simulink model "G2V"  (R2017a)
settings: Solver=ode23t  StartTime=0.0  StopTime=10  RelTol=1e-3
values from neighbouring files (symbols this model uses):
  C_Vdc = 100*18e-3    (= 1.8)    [main_v2gg2v.m]
  Cf = 10*165e-6    (= 0.00165)    [main_v2gg2v.m]
  D = 20    [main_v2gg2v.m]
  E1 = 1.07364213042869    (= 1.07364213043)    [main_v2gg2v.m]
  E2 = 1.05726676017896    (= 1.05726676018)    [main_v2gg2v.m]
  E3 = 1.05298913370226    (= 1.0529891337)    [main_v2gg2v.m]
  f_grid = 50    [main_v2gg2v.m]
  H1 = 10    [main_v2gg2v.m]
  H2 = 15    [main_v2gg2v.m]
  H3 = 60    [main_v2gg2v.m]
  h_PEV = -2000    [main_v2gg2v.m]
  Ibat_ref = -200    [main_v2gg2v.m]
  Ibatfault_ref = 200    [main_v2gg2v.m]
  Ki_CC = 1    [main_v2gg2v.m]
  Ki_inner = 5000    [main_v2gg2v.m]
  Ki_outer = 10000    [main_v2gg2v.m]
  Ki_PLL = 10000    [main_v2gg2v.m]
  Kp_CC = 10    [main_v2gg2v.m]
  Kp_inner = 100    [main_v2gg2v.m]
  Kp_outer = 250    [main_v2gg2v.m]
  Kp_PLL = 100    [main_v2gg2v.m]
  Lbat = 2e-3    (= 0.002)    [main_v2gg2v.m]
  Lgrid = 1/10*0.69e-3    (= 6.9e-05)    [main_v2gg2v.m]
  Linv = 1/10*0.48e-3    (= 4.8e-05)    [main_v2gg2v.m]
  LowSat_CC = 0    [main_v2gg2v.m]
  omega = 2*pi*f_grid    (= 314.159265359)    [main_v2gg2v.m]
  Pm1 = 2.49    [main_v2gg2v.m]
  Pm2 = 4.21    [main_v2gg2v.m]
  Pm3 = 8.20    (= 8.2)    [main_v2gg2v.m]
  Rd = 1.31    [main_v2gg2v.m]
  S1pu = (1.5 + .45j)    [main_v2gg2v.m]
  S2pu = (1.0 + .3j)    [main_v2gg2v.m]
  S3pu = (12.4 + 2.5j)    [main_v2gg2v.m]
  Sbase = 1e6    (= 1000000)    [main_v2gg2v.m]
  Snom_trafo = 1050e6    (= 1050000000)    [main_v2gg2v.m]
  t_fault_end = t_fault_start + FCT    (= 0.723)    [main_v2gg2v.m]
  t_fault_start = 0.5    [main_v2gg2v.m]
  Ts = 1e-5    (= 1e-05)    [main_v2gg2v.m]
  UpSat_CC = 1    [main_v2gg2v.m]
  Vbase = 345e3    (= 345000)    [main_v2gg2v.m]
  Vdc_ref = 1.5e3    (= 1500)    [main_v2gg2v.m]
  Vfault_thresh = 455    [main_v2gg2v.m]
undefined symbols (not defined in the file or in its folder): D1, Delta, Ion, L12, L13, L23, Lbuckboost, Lithium, R_Vdc, Rbuckboost
libraries: powerlib x175, powerlib_meascontrol x55, simulink x45, electricdrivelib x30, dspstat3 x3
(part 1 of 5)
settings Model: Creator=BagaskaraPP  LastModifiedBy=BagaskaraPP
settings SolverCC: ZeroCrossAlgorithm=Adaptive
settings DataIOCC: Refine=4
settings DebuggingCC: MaxConsecutiveZCsMsg=none

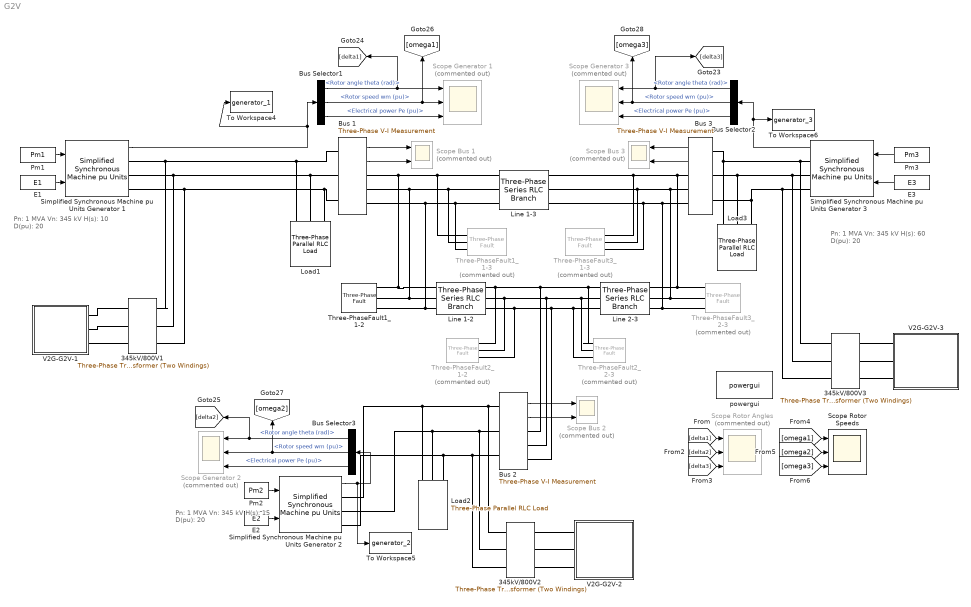
== system G2V ==
  note: Pn: 1 MVA
      | Vn: 345 kV
      | H(s): 15
      | D(pu): 20
  note: Pn: 1 MVA
      | Vn: 345 kV
      | H(s): 60
      | D(pu): 20
  note: Pn: 1 MVA
      | Vn: 345 kV
      | H(s): 10
      | D(pu): 20
  345kV/800V1 : powerlib/Elements/Three-Phase Transformer (Two Windings)  Winding1Connection=Delta (D1)  Winding2Connection=Yg  CoreType=Three single-phase transformers  SetSaturation=off  Hysteresis=off  DataFile='hysteresis'  SetInitialFlux=off  Measurements=None  UNITS=pu  NominalPower=[ Snom_trafo , f_grid ]  Winding1=[Vbase , 0 , 0 ]  Winding2=[ 800 , 0 , 0 ]  Rm=0  Lm=0  L0=0.5  Saturation=[ 0,0 ; 0.0024,1.2 ; 1.0,1.52 ]  InitialFluxes=[ 0.8 , -0.8 , 0.7 ]  MoreParameters=off  BreakLoop=off  DataType=off  TransfoNumber=1
  345kV/800V2 : powerlib/Elements/Three-Phase Transformer (Two Windings)  Winding1Connection=Delta (D1)  Winding2Connection=Yg  CoreType=Three single-phase transformers  SetSaturation=off  Hysteresis=off  DataFile='hysteresis'  SetInitialFlux=off  Measurements=None  UNITS=pu  NominalPower=[ Snom_trafo , f_grid ]  Winding1=[Vbase , 0 , 0 ]  Winding2=[ 800 , 0 , 0 ]  Rm=0  Lm=0  L0=0.5  Saturation=[ 0,0 ; 0.0024,1.2 ; 1.0,1.52 ]  InitialFluxes=[ 0.8 , -0.8 , 0.7 ]  MoreParameters=off  BreakLoop=off  DataType=off  TransfoNumber=1
  345kV/800V3 : powerlib/Elements/Three-Phase Transformer (Two Windings)  Winding1Connection=Delta (D1)  Winding2Connection=Yg  CoreType=Three single-phase transformers  SetSaturation=off  Hysteresis=off  DataFile='hysteresis'  SetInitialFlux=off  Measurements=None  UNITS=pu  NominalPower=[ Snom_trafo , f_grid ]  Winding1=[Vbase , 0 , 0 ]  Winding2=[ 800 , 0 , 0 ]  Rm=0  Lm=0  L0=0.5  Saturation=[ 0,0 ; 0.0024,1.2 ; 1.0,1.52 ]  InitialFluxes=[ 0.8 , -0.8 , 0.7 ]  MoreParameters=off  BreakLoop=off  DataType=off  TransfoNumber=1
  Bus Selector1 : BusSelector  OutputSignals=Rotor angle theta (rad),Rotor speed wm (pu),Electrical power Pe (pu)
  Bus Selector2 : BusSelector  OutputSignals=Rotor angle theta (rad),Rotor speed wm (pu),Electrical power Pe (pu)
  Bus Selector3 : BusSelector  OutputSignals=Rotor angle theta (rad),Rotor speed wm (pu),Electrical power Pe (pu)
  Bus 1 : powerlib/Measurements/Three-Phase V-I Measurement  VoltageMeasurement=phase-to-ground  SetLabelV=off  LabelV=Vabc  Vpu=off  VpuLL=off  CurrentMeasurement=yes  SetLabelI=off  LabelI=Iabc  Ipu=off  Pbase=100e6  Vbase=500e3  OutputType=Complex  PhasorSimulation=off  PSBequivalent=0
  Bus 2 : powerlib/Measurements/Three-Phase V-I Measurement  VoltageMeasurement=phase-to-ground  SetLabelV=off  LabelV=Vabc  Vpu=off  VpuLL=off  CurrentMeasurement=yes  SetLabelI=off  LabelI=Iabc  Ipu=off  Pbase=100e6  Vbase=500e3  OutputType=Complex  PhasorSimulation=off  PSBequivalent=0
  Bus 3 : powerlib/Measurements/Three-Phase V-I Measurement  VoltageMeasurement=phase-to-ground  SetLabelV=off  LabelV=Vabc  Vpu=off  VpuLL=off  CurrentMeasurement=yes  SetLabelI=off  LabelI=Iabc  Ipu=off  Pbase=100e6  Vbase=500e3  OutputType=Complex  PhasorSimulation=off  PSBequivalent=0
  E1 : Constant  Value=E1
  E2 : Constant  Value=E2
  E3 : Constant  Value=E3
  Line 1-2 : powerlib/Elements/Three-Phase Series RLC Branch  LConnTagsString=A|B|C  RConnTagsString=A|B|C  BranchType=RL  Resistance=0  Inductance=L12  Capacitance=1e-6  Measurements=None
  Line 1-3 : powerlib/Elements/Three-Phase Series RLC Branch  LConnTagsString=A|B|C  RConnTagsString=A|B|C  BranchType=RL  Resistance=0  Inductance=L13  Capacitance=1e-6  Measurements=None
  Line 2-3 : powerlib/Elements/Three-Phase Series RLC Branch  LConnTagsString=A|B|C  RConnTagsString=A|B|C  BranchType=RL  Resistance=0  Inductance=L23  Capacitance=1e-6  Measurements=None
  Load1 : powerlib/Elements/Three-Phase Parallel RLC Load  LConnTagsString=A|B|C  Configuration=Y (grounded)  NominalVoltage=Vbase  Vabc=[1e3 1e3 1e3]  Vabcp=[1e3 1e3 1e3]  NominalFrequency=f_grid  UnbalancedPower=off  ActivePower=real(S1pu)*Sbase  InductivePower=imag(S1pu)*Sbase  CapacitivePower=0  Pabc=[10e3 9e3 11e3]  QLabc=[100 90 110]  QCabc=[100 90 110]  Pabcp=[10e3 9e3 11e3]  QLabcp=[100 90 110]  QCabcp=[100 90 110]  Measurements=None  LoadType=constant PQ
  Load2 : powerlib/Elements/Three-Phase Parallel RLC Load  LConnTagsString=A|B|C  Configuration=Y (grounded)  NominalVoltage=Vbase  Vabc=[1e3 1e3 1e3]  Vabcp=[1e3 1e3 1e3]  NominalFrequency=f_grid  UnbalancedPower=off  ActivePower=real(S2pu)*Sbase  InductivePower=imag(S2pu)*Sbase  CapacitivePower=0  Pabc=[10e3 9e3 11e3]  QLabc=[100 90 110]  QCabc=[100 90 110]  Pabcp=[10e3 9e3 11e3]  QLabcp=[100 90 110]  QCabcp=[100 90 110]  Measurements=None  LoadType=constant PQ
  Load3 : powerlib/Elements/Three-Phase Parallel RLC Load  LConnTagsString=A|B|C  Configuration=Y (grounded)  NominalVoltage=Vbase  Vabc=[1e3 1e3 1e3]  Vabcp=[1e3 1e3 1e3]  NominalFrequency=f_grid  UnbalancedPower=off  ActivePower=real(S3pu)*Sbase  InductivePower=imag(S3pu)*Sbase  CapacitivePower=0  Pabc=[10e3 9e3 11e3]  QLabc=[100 90 110]  QCabc=[100 90 110]  Pabcp=[10e3 9e3 11e3]  QLabcp=[100 90 110]  QCabcp=[100 90 110]  Measurements=None  LoadType=constant PQ
  Pm1 : Constant  Value=Pm1
  Pm2 : Constant  Value=Pm2
  Pm3 : Constant  Value=Pm3
  Scope Bus 1 : Scope  Commented=on  NumInputPorts=2
  Scope Bus 2 : Scope  Commented=on  NumInputPorts=2
  Scope Bus 3 : Scope  Commented=on  NumInputPorts=2
  Scope Generator 1 : Scope  Commented=on  NumInputPorts=3
  Scope Generator 2 : Scope  Commented=on  NumInputPorts=3
  Scope Generator 3 : Scope  Commented=on  NumInputPorts=3
  Scope Rotor Angles : Scope  Commented=on  NumInputPorts=3
  Scope Rotor Speeds : Scope  NumInputPorts=3
  Simplified Synchronous Machine pu Units Generator 1 : powerlib/Machines/Simplified Synchronous Machine pu Units  ConnectionType=3-wire Y  MechanicalLoad=Mechanical power Pm  MeasurementBus=off  NominalParameters=[Sbase Vbase f_grid]  Mechanical=[H1 D 1]  InternalRL="[0.0  0.088]"  InitialConditions="[ 0,26.7181   2.5567,2.5567,2.5567   15,15-120,15+120 ]"  Units=0  LoadFlowParameters=[1,0,0,0,0]  TsPowergui=0  TsBlock=-1  BusType=PV  Pref=0  Qref=0  Qmin=-inf  Qmax=+inf  PLF=0  QLF=0
      settings: SourceProductName=Simscape Power Systems  SourceProductBaseCode=PS
  Simplified Synchronous Machine pu Units Generator 2 : powerlib/Machines/Simplified Synchronous Machine pu Units  ConnectionType=3-wire Y  MechanicalLoad=Mechanical power Pm  MeasurementBus=off  NominalParameters=[Sbase Vbase f_grid]  Mechanical=[H2 D 1]  InternalRL="[0.0  0.05]"  InitialConditions="[ 0,26.4706   4.2715,4.2715,4.2715   15,15-120,15+120 ]"  Units=0  LoadFlowParameters=[1,0,0,0,0]  TsPowergui=0  TsBlock=-1  BusType=PV  Pref=0  Qref=0  Qmin=-inf  Qmax=+inf  PLF=0  QLF=0
      settings: SourceProductName=Simscape Power Systems  SourceProductBaseCode=PS
  Simplified Synchronous Machine pu Units Generator 3 : powerlib/Machines/Simplified Synchronous Machine pu Units  ConnectionType=3-wire Y  MechanicalLoad=Mechanical power Pm  MeasurementBus=off  NominalParameters=[Sbase Vbase f_grid]  Mechanical=[H3 D 1]  InternalRL="[0.0  0.015]"  InitialConditions="[ 0,6.7081   8.7496,8.7496,8.7496   0,-120,120 ]"  Units=0  LoadFlowParameters=[1,0,0,0,0]  TsPowergui=0  TsBlock=-1  BusType=PV  Pref=0  Qref=0  Qmin=-inf  Qmax=+inf  PLF=0  QLF=0
      settings: SourceProductName=Simscape Power Systems  SourceProductBaseCode=PS
  Three-PhaseFault1_1-2 : powerlib/Elements/Three-Phase Fault  InitialStates=0  FaultA=on  FaultB=on  FaultC=on  GroundFault=on  SwitchTimes="[t_fault_start  t_fault_end]"  External=off  SwitchStatus=NaN  FaultResistance=0.001  GroundResistance=0.01  SnubberResistance=1e6  SnubberCapacitance=inf  Measurements=None
  Three-PhaseFault1_1-3 : powerlib/Elements/Three-Phase Fault  Commented=on  InitialStates=0  FaultA=on  FaultB=on  FaultC=on  GroundFault=on  SwitchTimes="[t_fault_start  t_fault_end]"  External=off  SwitchStatus=NaN  FaultResistance=0.001  GroundResistance=0.01  SnubberResistance=1e6  SnubberCapacitance=inf  Measurements=None
  Three-PhaseFault2_1-2 : powerlib/Elements/Three-Phase Fault  Commented=on  InitialStates=0  FaultA=on  FaultB=on  FaultC=on  GroundFault=on  SwitchTimes="[t_fault_start  t_fault_end]"  External=off  SwitchStatus=NaN  FaultResistance=0.001  GroundResistance=0.01  SnubberResistance=1e6  SnubberCapacitance=inf  Measurements=None
  Three-PhaseFault2_2-3 : powerlib/Elements/Three-Phase Fault  Commented=on  InitialStates=0  FaultA=on  FaultB=on  FaultC=on  GroundFault=on  SwitchTimes="[t_fault_start  t_fault_end]"  External=off  SwitchStatus=NaN  FaultResistance=0.001  GroundResistance=0.01  SnubberResistance=1e6  SnubberCapacitance=inf  Measurements=None
  Three-PhaseFault3_1-3 : powerlib/Elements/Three-Phase Fault  Commented=on  InitialStates=0  FaultA=on  FaultB=on  FaultC=on  GroundFault=on  SwitchTimes="[t_fault_start  t_fault_end]"  External=off  SwitchStatus=NaN  FaultResistance=0.001  GroundResistance=0.01  SnubberResistance=1e6  SnubberCapacitance=inf  Measurements=None
  Three-PhaseFault3_2-3 : powerlib/Elements/Three-Phase Fault  Commented=on  InitialStates=0  FaultA=on  FaultB=on  FaultC=on  GroundFault=on  SwitchTimes="[t_fault_start  t_fault_end]"  External=off  SwitchStatus=NaN  FaultResistance=0.001  GroundResistance=0.01  SnubberResistance=1e6  SnubberCapacitance=inf  Measurements=None
  To Workspace4 : ToWorkspace  VariableName=generator_1  SaveFormat=Timeseries  SampleTime=-1
  To Workspace5 : ToWorkspace  VariableName=generator_2  SaveFormat=Timeseries  SampleTime=-1
  To Workspace6 : ToWorkspace  VariableName=generator_3  SaveFormat=Timeseries  SampleTime=-1
  V2G-G2V-1 : Subsystem
  V2G-G2V-2 : Subsystem
  V2G-G2V-3 : Subsystem
  powergui : powerlib/powergui  Priority=1  SimulationMode=Discrete  SampleTime=Ts  frequency=60  Iterations=50  frequencyindice=0  Pbase=100e6  ErrMax=1e-4  UnitsV=kV  UnitsW=MW  buscounter=0  FunctionMessages=off  echomessages=off  EnableUseOfTLC=off  CurrentSourceSwitches=off  DisableSnubberDevices=off  DisableRonSwitches=off  DisableVfSwitches=off  DisplayEquations=off  SolverType=Tustin/Backward Euler (TBE)  Interpol=off  ExternalGateDelay=off  methode=off  Ts=100  x0status=blocks  SPID=on  SwTol=0  HookPort=off  RestoreLinks=warning  ResistiveCurrentMeasurement=off  Frange=[0:2:500]  Ylog=off  Xlog=on  ShowGrid=off  save=off  variable=ZData  structure=0  ZoomFFT=off  StartTime=0.0  cycles=1  DisplayStyle=1  fundamental=60  FreqAxis=off  MaxFrequency=1000  frequencyindicesteady=1  RmsSteady=1  display=off
  wires:
  Bus 1/1 -> Scope Bus 1/1
  Pm2/1 -> Simplified Synchronous Machine pu Units Generator 2/1
  Bus Selector2/2 -> [omega3], Scope Generator 3/2  "<Rotor speed wm (pu)>"
  Bus Selector2/1 -> Scope Generator 3/1, [delta3]  "<Rotor angle theta (rad)>"
  Pm3/1 -> Simplified Synchronous Machine pu Units Generator 3/1
  Bus 2/2 -> Scope Bus 2/2
  Bus Selector3/3 -> Scope Generator 2/3  "<Electrical power Pe (pu)>"
  Bus Selector2/3 -> Scope Generator 3/3  "<Electrical power Pe (pu)>"
  Bus 1/2 -> Scope Bus 1/2
  Bus Selector3/2 -> Scope Generator 2/2, [omega2]  "<Rotor speed wm (pu)>"
  Bus 3/2 -> Scope Bus 3/2
  Bus Selector3/1 -> Scope Generator 2/1, [delta2]  "<Rotor angle theta (rad)>"
  Bus 3/1 -> Scope Bus 3/1
  Bus 2/1 -> Scope Bus 2/1
  E1/1 -> Simplified Synchronous Machine pu Units Generator 1/2
  Pm1/1 -> Simplified Synchronous Machine pu Units Generator 1/1
  Simplified Synchronous Machine pu Units Generator 1/1 -> To Workspace4/1, Bus Selector1/1
  Bus Selector1/3 -> Scope Generator 1/3  "<Electrical power Pe (pu)>"
  Simplified Synchronous Machine pu Units Generator 3/1 -> To Workspace6/1, Bus Selector2/1
  Bus Selector1/2 -> Scope Generator 1/2, [omega1]  "<Rotor speed wm (pu)>"
  Bus Selector1/1 -> Scope Generator 1/1, [delta1]  "<Rotor angle theta (rad)>"
  Simplified Synchronous Machine pu Units Generator 2/1 -> To Workspace5/1, Bus Selector3/1
  E2/1 -> Simplified Synchronous Machine pu Units Generator 2/2
  E3/1 -> Simplified Synchronous Machine pu Units Generator 3/2
  [omega2] -> Scope Rotor Speeds/2
  [delta2] -> Scope Rotor Angles/2
  [delta3] -> Scope Rotor Angles/3
  [delta1] -> Scope Rotor Angles/1
  [omega3] -> Scope Rotor Speeds/3
  [omega1] -> Scope Rotor Speeds/1
  connections:
  Line 1-2/LConn1 -- Three-PhaseFault1_1-2/LConn1 -- Three-PhaseFault1_1-3/LConn1 -- Line 1-3/LConn1 -- Bus 1/RConn1
  Load1/LConn3 -- 345kV/800V1/LConn3 -- Simplified Synchronous Machine pu Units Generator 1/RConn3 -- Bus 1/LConn3
  Three-PhaseFault2_1-2/LConn2 -- Line 1-2/RConn2 -- Bus 2/RConn2 -- Three-PhaseFault2_2-3/LConn2 -- Line 2-3/LConn2
  Load3/LConn3 -- 345kV/800V3/LConn3 -- Simplified Synchronous Machine pu Units Generator 3/RConn3 -- Bus 3/LConn3
  Load2/LConn2 -- 345kV/800V2/LConn2 -- Bus 2/LConn2 -- Simplified Synchronous Machine pu Units Generator 2/RConn2
  Bus 3/RConn2 -- Three-PhaseFault3_2-3/LConn2 -- Line 2-3/RConn2 -- Line 1-3/RConn2 -- Three-PhaseFault3_1-3/LConn2
  Bus 3/RConn3 -- Three-PhaseFault3_2-3/LConn3 -- Line 2-3/RConn3 -- Line 1-3/RConn3 -- Three-PhaseFault3_1-3/LConn3
  Load1/LConn2 -- 345kV/800V1/LConn2 -- Simplified Synchronous Machine pu Units Generator 1/RConn2 -- Bus 1/LConn2
  Simplified Synchronous Machine pu Units Generator 2/RConn1 -- Load2/LConn1 -- 345kV/800V2/LConn1 -- Bus 2/LConn1
  Load3/LConn1 -- 345kV/800V3/LConn1 -- Simplified Synchronous Machine pu Units Generator 3/RConn1 -- Bus 3/LConn1
  Line 2-3/LConn1 -- Three-PhaseFault2_2-3/LConn1 -- Bus 2/RConn1 -- Three-PhaseFault2_1-2/LConn1 -- Line 1-2/RConn1
  Load3/LConn2 -- 345kV/800V3/LConn2 -- Simplified Synchronous Machine pu Units Generator 3/RConn2 -- Bus 3/LConn2
  Line 1-3/RConn1 -- Three-PhaseFault3_1-3/LConn1 -- Three-PhaseFault3_2-3/LConn1 -- Line 2-3/RConn1 -- Bus 3/RConn1
  Load2/LConn3 -- Simplified Synchronous Machine pu Units Generator 2/RConn3 -- 345kV/800V2/LConn3 -- Bus 2/LConn3
  Line 1-3/LConn2 -- Three-PhaseFault1_1-3/LConn2 -- Line 1-2/LConn2 -- Three-PhaseFault1_1-2/LConn2 -- Bus 1/RConn2
  Line 1-2/LConn3 -- Three-PhaseFault1_1-3/LConn3 -- Line 1-3/LConn3 -- Bus 1/RConn3 -- Three-PhaseFault1_1-2/LConn3
  Bus 1/LConn1 -- 345kV/800V1/LConn1 -- Simplified Synchronous Machine pu Units Generator 1/RConn1 -- Load1/LConn1
  Three-PhaseFault2_1-2/LConn3 -- Line 1-2/RConn3 -- Bus 2/RConn3 -- Three-PhaseFault2_2-3/LConn3 -- Line 2-3/LConn3
  345kV/800V2/RConn1 -- V2G-G2V-2/LConn1
  345kV/800V2/RConn2 -- V2G-G2V-2/LConn2
  345kV/800V2/RConn3 -- V2G-G2V-2/LConn3
  V2G-G2V-1/LConn1 -- 345kV/800V1/RConn1
  V2G-G2V-1/LConn2 -- 345kV/800V1/RConn2
  V2G-G2V-1/LConn3 -- 345kV/800V1/RConn3
  V2G-G2V-3/LConn1 -- 345kV/800V3/RConn1
  V2G-G2V-3/LConn2 -- 345kV/800V3/RConn2
  V2G-G2V-3/LConn3 -- 345kV/800V3/RConn3

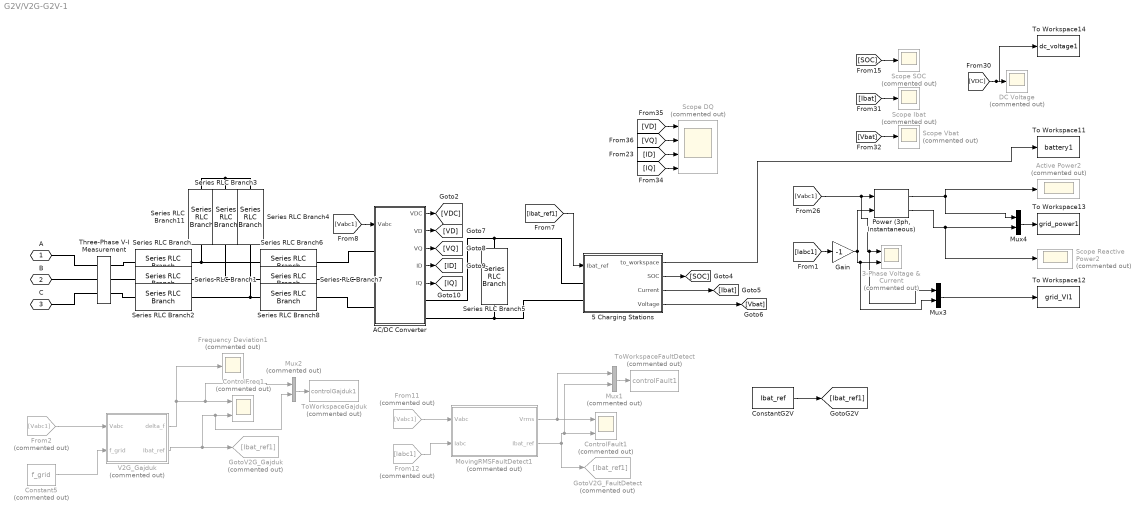
== system G2V/V2G-G2V-1 ==
  3-Phase Voltage & Current : Scope  Commented=on  NumInputPorts=2
  5 Charging Stations : Subsystem
  AC/DC Converter : Subsystem
  Active Power2 : Scope  Commented=on
  Constant5 : Constant  Commented=on  Value=f_grid
  ConstantG2V : Constant  Value=Ibat_ref
  ControlFault1 : Scope  Commented=on  NumInputPorts=2
  ControlFreq1 : Scope  Commented=on  NumInputPorts=2
  DC Voltage : Scope  Commented=on
  Frequency Deviation1 : Scope  Commented=on
  From11 : From  Commented=on  GotoTag=Vabc1  TagVisibility=global
  From12 : From  Commented=on  GotoTag=Iabc1  TagVisibility=global
  From2 : From  Commented=on  GotoTag=Vabc1  TagVisibility=global
  Gain : Gain  Gain=-1
  GotoV2G_FaultDetect : Goto  Commented=on  GotoTag=Ibat_ref1
  GotoV2G_Gajduk : Goto  Commented=on  GotoTag=Ibat_ref1
  MovingRMSFaultDetect1 : Subsystem  Commented=on
  Mux1 : Mux  Commented=on  Inputs=2
  Mux2 : Mux  Commented=on  Inputs=2
  Mux3 : Mux  Inputs=2
  Mux4 : Mux  Inputs=2
  "Power (3ph, Instantaneous)" : powerlib_meascontrol/Measurements/Power (3ph, Instantaneous)
      settings: SourceProductName=Simscape Power Systems
  Scope DQ : Scope  Commented=on  NumInputPorts=4
  Scope Ibat : Scope  Commented=on
  Scope Reactive Power2 : Scope  Commented=on
  Scope SOC : Scope  Commented=on
  Scope Vbat : Scope  Commented=on
  Series RLC Branch : powerlib/Elements/Series RLC Branch  LConnTagsString=__new0  RConnTagsString=__new0  BranchType=L  Resistance=1  Inductance=Lgrid  SetiL0=off  InitialCurrent=0  Capacitance=1e-6  Setx0=off  InitialVoltage=0  Measurements=None
  Series RLC Branch1 : powerlib/Elements/Series RLC Branch  LConnTagsString=__new0  RConnTagsString=__new0  BranchType=L  Resistance=1  Inductance=Lgrid  SetiL0=off  InitialCurrent=0  Capacitance=1e-6  Setx0=off  InitialVoltage=0  Measurements=None
  Series RLC Branch11 : powerlib/Elements/Series RLC Branch  LConnTagsString=__new0  RConnTagsString=__new0  BranchType=RC  Resistance=Rd  Inductance=Lbuckboost  SetiL0=off  InitialCurrent=0  Capacitance=Cf  Setx0=off  InitialVoltage=0  Measurements=None
  Series RLC Branch2 : powerlib/Elements/Series RLC Branch  LConnTagsString=__new0  RConnTagsString=__new0  BranchType=L  Resistance=1  Inductance=Lgrid  SetiL0=off  InitialCurrent=0  Capacitance=1e-6  Setx0=off  InitialVoltage=0  Measurements=None
  Series RLC Branch3 : powerlib/Elements/Series RLC Branch  LConnTagsString=__new0  RConnTagsString=__new0  BranchType=RC  Resistance=Rd  Inductance=Lbuckboost  SetiL0=off  InitialCurrent=0  Capacitance=Cf  Setx0=off  InitialVoltage=0  Measurements=None
  Series RLC Branch4 : powerlib/Elements/Series RLC Branch  LConnTagsString=__new0  RConnTagsString=__new0  BranchType=RC  Resistance=Rd  Inductance=Lbuckboost  SetiL0=off  InitialCurrent=0  Capacitance=Cf  Setx0=off  InitialVoltage=0  Measurements=None
  Series RLC Branch5 : powerlib/Elements/Series RLC Branch  LConnTagsString=__new0  RConnTagsString=__new0  BranchType=C  Resistance=R_Vdc  Inductance=1e-3  SetiL0=off  InitialCurrent=0  Capacitance=C_Vdc  Setx0=on  InitialVoltage=V0_Vdc  Measurements=None
  Series RLC Branch6 : powerlib/Elements/Series RLC Branch  LConnTagsString=__new0  RConnTagsString=__new0  BranchType=L  Resistance=1  Inductance=Linv  SetiL0=off  InitialCurrent=0  Capacitance=1e-6  Setx0=off  InitialVoltage=0  Measurements=None
  Series RLC Branch7 : powerlib/Elements/Series RLC Branch  LConnTagsString=__new0  RConnTagsString=__new0  BranchType=L  Resistance=1  Inductance=Linv  SetiL0=off  InitialCurrent=0  Capacitance=1e-6  Setx0=off  InitialVoltage=0  Measurements=None
  Series RLC Branch8 : powerlib/Elements/Series RLC Branch  LConnTagsString=__new0  RConnTagsString=__new0  BranchType=L  Resistance=1  Inductance=Linv  SetiL0=off  InitialCurrent=0  Capacitance=1e-6  Setx0=off  InitialVoltage=0  Measurements=None
  Three-Phase V-I Measurement : powerlib/Measurements/Three-Phase V-I Measurement  VoltageMeasurement=phase-to-ground  SetLabelV=on  LabelV=Vabc1  Vpu=off  VpuLL=off  CurrentMeasurement=yes  SetLabelI=on  LabelI=Iabc1  Ipu=off  Pbase=100e6  Vbase=500e3  OutputType=Complex  PhasorSimulation=off  PSBequivalent=0
  To Workspace11 : ToWorkspace  VariableName=battery1  SaveFormat=Timeseries  SampleTime=-1
  To Workspace12 : ToWorkspace  VariableName=grid_VI1  SaveFormat=Timeseries  SampleTime=-1
  To Workspace13 : ToWorkspace  VariableName=grid_power1  SaveFormat=Timeseries  SampleTime=-1
  To Workspace14 : ToWorkspace  VariableName=dc_voltage1  SaveFormat=Timeseries  SampleTime=-1
  ToWorkspaceFaultDetect : ToWorkspace  Commented=on  VariableName=controlFault1  SaveFormat=Timeseries  SampleTime=-1
  ToWorkspaceGajduk : ToWorkspace  Commented=on  VariableName=controlGajduk1  SaveFormat=Timeseries  SampleTime=-1
  V2G_Gajduk : Subsystem  Commented=on
  A : PMIOPort  Port=1  Side=Left
  B : PMIOPort  Port=2  Side=Left
  C : PMIOPort  Port=3  Side=Left
  wires:
  AC/DC Converter/3(VQ) -> [VQ]
  [Iabc1] -> Gain/1
  [ID] -> Scope DQ/3
  AC/DC Converter/1(VDC) -> [VDC]
  AC/DC Converter/4(ID) -> [ID]
  [Ibat] -> Scope Ibat/1
  Gain/1 -> Mux3/2, 3-Phase Voltage & Current/2, "Power (3ph, Instantaneous)"/2
  AC/DC Converter/2(VD) -> [VD]
  [IQ] -> Scope DQ/4
  [VD] -> Scope DQ/1
  [VQ] -> Scope DQ/2
  [Ibat_ref1] -> 5 Charging Stations/1(Ibat_ref)
  5 Charging Stations/2(SOC) -> [SOC]
  5 Charging Stations/3(Current) -> [Ibat]
  [Vbat] -> Scope Vbat/1
  5 Charging Stations/4(Voltage) -> [Vbat]
  [Vabc1] -> Mux3/1, 3-Phase Voltage & Current/1, "Power (3ph, Instantaneous)"/1
  AC/DC Converter/5(IQ) -> [IQ]
  [Vabc1] -> AC/DC Converter/1(Vabc)
  [SOC] -> Scope SOC/1
  Mux4/1 -> To Workspace13/1
  "Power (3ph, Instantaneous)"/2 -> Scope Reactive Power2/1, Mux4/2
  [VDC] -> To Workspace14/1, DC Voltage/1
  Mux3/1 -> To Workspace12/1
  "Power (3ph, Instantaneous)"/1 -> Mux4/1, Active Power2/1
  5 Charging Stations/1(to_workspace) -> To Workspace11/1
  V2G_Gajduk/2(Ibat_ref) -> Mux2/2, ControlFreq1/2, GotoV2G_Gajduk/1
  V2G_Gajduk/1(delta_f) -> Mux2/1, ControlFreq1/1, Frequency Deviation1/1
  Constant5/1 -> V2G_Gajduk/2(f_grid)
  Mux2/1 -> ToWorkspaceGajduk/1
  From2/1 -> V2G_Gajduk/1(Vabc)
  Mux1/1 -> ToWorkspaceFaultDetect/1
  From12/1 -> MovingRMSFaultDetect1/2(Iabc)
  MovingRMSFaultDetect1/1(Vrms) -> Mux1/1, ControlFault1/1
  From11/1 -> MovingRMSFaultDetect1/1(Vabc)
  MovingRMSFaultDetect1/2(Ibat_ref) -> Mux1/2, ControlFault1/2, GotoV2G_FaultDetect/1
  ConstantG2V/1 -> [Ibat_ref1]
  connections:
  Series RLC Branch5/LConn1 -- 5 Charging Stations/LConn1 -- AC/DC Converter/RConn1
  Series RLC Branch6/LConn1 -- Series RLC Branch11/LConn1 -- Series RLC Branch/RConn1
  Series RLC Branch4/LConn1 -- Series RLC Branch8/LConn1 -- Series RLC Branch2/RConn1
  B/RConn1 -- Three-Phase V-I Measurement/LConn2
  Series RLC Branch/LConn1 -- Three-Phase V-I Measurement/RConn1
  A/RConn1 -- Three-Phase V-I Measurement/LConn1
  AC/DC Converter/LConn1 -- Series RLC Branch6/RConn1
  AC/DC Converter/LConn3 -- Series RLC Branch8/RConn1
  Series RLC Branch3/LConn1 -- Series RLC Branch1/RConn1 -- Series RLC Branch7/LConn1
  Series RLC Branch1/LConn1 -- Three-Phase V-I Measurement/RConn2
  5 Charging Stations/LConn2 -- Series RLC Branch5/RConn1 -- AC/DC Converter/RConn2
  Series RLC Branch11/RConn1 -- Series RLC Branch4/RConn1 -- Series RLC Branch3/RConn1
  C/RConn1 -- Three-Phase V-I Measurement/LConn3
  AC/DC Converter/LConn2 -- Series RLC Branch7/RConn1
  Series RLC Branch2/LConn1 -- Three-Phase V-I Measurement/RConn3

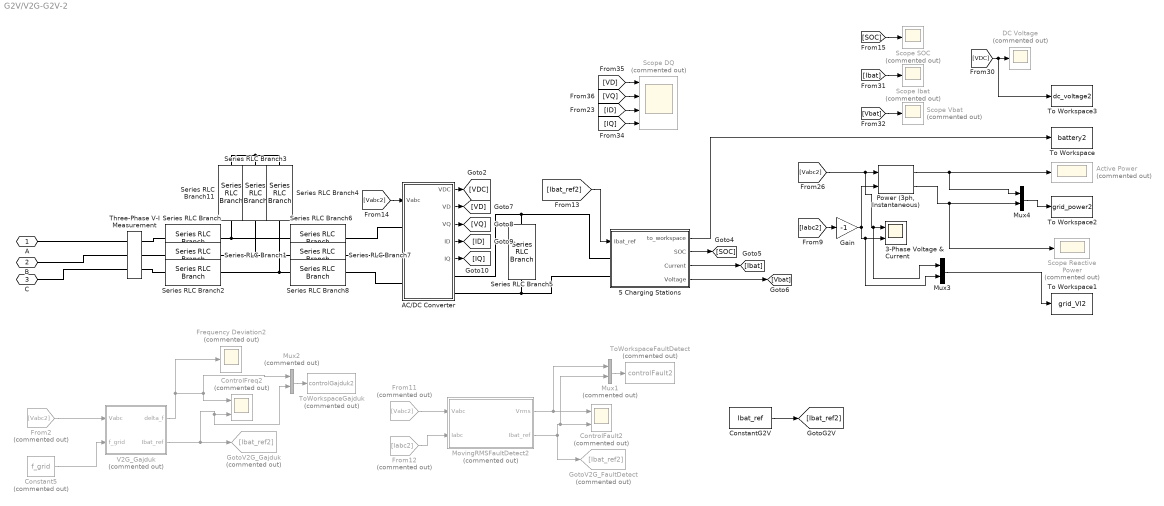
== system G2V/V2G-G2V-2 ==
  3-Phase Voltage & Current : Scope  NumInputPorts=2
  5 Charging Stations : Subsystem
  AC/DC Converter : Subsystem
  Active Power : Scope  Commented=on
  Constant5 : Constant  Commented=on  Value=f_grid
  ConstantG2V : Constant  Value=Ibat_ref
  ControlFault2 : Scope  Commented=on  NumInputPorts=2
  ControlFreq2 : Scope  Commented=on  NumInputPorts=2
  DC Voltage : Scope  Commented=on
  Frequency Deviation2 : Scope  Commented=on
  From11 : From  Commented=on  GotoTag=Vabc2  TagVisibility=global
  From12 : From  Commented=on  GotoTag=Iabc2  TagVisibility=global
  From2 : From  Commented=on  GotoTag=Vabc2  TagVisibility=global
  Gain : Gain  Gain=-1
  GotoV2G_FaultDetect : Goto  Commented=on  GotoTag=Ibat_ref2
  GotoV2G_Gajduk : Goto  Commented=on  GotoTag=Ibat_ref2
  MovingRMSFaultDetect2 : Subsystem  Commented=on
  Mux1 : Mux  Commented=on  Inputs=2
  Mux2 : Mux  Commented=on  Inputs=2
  Mux3 : Mux  Inputs=2
  Mux4 : Mux  Inputs=2
  "Power (3ph, Instantaneous)" : powerlib_meascontrol/Measurements/Power (3ph, Instantaneous)
      settings: SourceProductName=Simscape Power Systems
  Scope DQ : Scope  Commented=on  NumInputPorts=4
  Scope Ibat : Scope  Commented=on
  Scope Reactive Power : Scope  Commented=on
  Scope SOC : Scope  Commented=on
  Scope Vbat : Scope  Commented=on
  Series RLC Branch : powerlib/Elements/Series RLC Branch  LConnTagsString=__new0  RConnTagsString=__new0  BranchType=L  Resistance=1  Inductance=Lgrid  SetiL0=off  InitialCurrent=0  Capacitance=1e-6  Setx0=off  InitialVoltage=0  Measurements=None
  Series RLC Branch1 : powerlib/Elements/Series RLC Branch  LConnTagsString=__new0  RConnTagsString=__new0  BranchType=L  Resistance=1  Inductance=Lgrid  SetiL0=off  InitialCurrent=0  Capacitance=1e-6  Setx0=off  InitialVoltage=0  Measurements=None
  Series RLC Branch11 : powerlib/Elements/Series RLC Branch  LConnTagsString=__new0  RConnTagsString=__new0  BranchType=RC  Resistance=Rd  Inductance=Lbuckboost  SetiL0=off  InitialCurrent=0  Capacitance=Cf  Setx0=off  InitialVoltage=0  Measurements=None
  Series RLC Branch2 : powerlib/Elements/Series RLC Branch  LConnTagsString=__new0  RConnTagsString=__new0  BranchType=L  Resistance=1  Inductance=Lgrid  SetiL0=off  InitialCurrent=0  Capacitance=1e-6  Setx0=off  InitialVoltage=0  Measurements=None
  Series RLC Branch3 : powerlib/Elements/Series RLC Branch  LConnTagsString=__new0  RConnTagsString=__new0  BranchType=RC  Resistance=Rd  Inductance=Lbuckboost  SetiL0=off  InitialCurrent=0  Capacitance=Cf  Setx0=off  InitialVoltage=0  Measurements=None
  Series RLC Branch4 : powerlib/Elements/Series RLC Branch  LConnTagsString=__new0  RConnTagsString=__new0  BranchType=RC  Resistance=Rd  Inductance=Lbuckboost  SetiL0=off  InitialCurrent=0  Capacitance=Cf  Setx0=off  InitialVoltage=0  Measurements=None
  Series RLC Branch5 : powerlib/Elements/Series RLC Branch  LConnTagsString=__new0  RConnTagsString=__new0  BranchType=C  Resistance=R_Vdc  Inductance=1e-3  SetiL0=off  InitialCurrent=0  Capacitance=C_Vdc  Setx0=on  InitialVoltage=V0_Vdc  Measurements=None
  Series RLC Branch6 : powerlib/Elements/Series RLC Branch  LConnTagsString=__new0  RConnTagsString=__new0  BranchType=L  Resistance=1  Inductance=Linv  SetiL0=off  InitialCurrent=0  Capacitance=1e-6  Setx0=off  InitialVoltage=0  Measurements=None
  Series RLC Branch7 : powerlib/Elements/Series RLC Branch  LConnTagsString=__new0  RConnTagsString=__new0  BranchType=L  Resistance=1  Inductance=Linv  SetiL0=off  InitialCurrent=0  Capacitance=1e-6  Setx0=off  InitialVoltage=0  Measurements=None
  Series RLC Branch8 : powerlib/Elements/Series RLC Branch  LConnTagsString=__new0  RConnTagsString=__new0  BranchType=L  Resistance=1  Inductance=Linv  SetiL0=off  InitialCurrent=0  Capacitance=1e-6  Setx0=off  InitialVoltage=0  Measurements=None
  Three-Phase V-I Measurement : powerlib/Measurements/Three-Phase V-I Measurement  VoltageMeasurement=phase-to-ground  SetLabelV=on  LabelV=Vabc2  Vpu=off  VpuLL=off  CurrentMeasurement=yes  SetLabelI=on  LabelI=Iabc2  Ipu=off  Pbase=100e6  Vbase=500e3  OutputType=Complex  PhasorSimulation=off  PSBequivalent=0
  To Workspace : ToWorkspace  VariableName=battery2  SaveFormat=Timeseries  SampleTime=-1
  To Workspace1 : ToWorkspace  VariableName=grid_VI2  SaveFormat=Timeseries  SampleTime=-1
  To Workspace2 : ToWorkspace  VariableName=grid_power2  SaveFormat=Timeseries  SampleTime=-1
  To Workspace3 : ToWorkspace  VariableName=dc_voltage2  SaveFormat=Timeseries  SampleTime=-1
  ToWorkspaceFaultDetect : ToWorkspace  Commented=on  VariableName=controlFault2  SaveFormat=Timeseries  SampleTime=-1
  ToWorkspaceGajduk : ToWorkspace  Commented=on  VariableName=controlGajduk2  SaveFormat=Timeseries  SampleTime=-1
  V2G_Gajduk : Subsystem  Commented=on
  A : PMIOPort  Port=1  Side=Left
  B : PMIOPort  Port=2  Side=Left
  C : PMIOPort  Port=3  Side=Left
  wires:
  [VQ] -> Scope DQ/2
  AC/DC Converter/2(VD) -> [VD]
  [Ibat_ref2] -> 5 Charging Stations/1(Ibat_ref)
  [Vabc2] -> AC/DC Converter/1(Vabc)
  5 Charging Stations/3(Current) -> [Ibat]
  AC/DC Converter/3(VQ) -> [VQ]
  [Iabc2] -> Gain/1
  [ID] -> Scope DQ/3
  [VD] -> Scope DQ/1
  AC/DC Converter/1(VDC) -> [VDC]
  [IQ] -> Scope DQ/4
  AC/DC Converter/4(ID) -> [ID]
  [SOC] -> Scope SOC/1
  Gain/1 -> Mux3/2, 3-Phase Voltage & Current/2, "Power (3ph, Instantaneous)"/2
  [Vbat] -> Scope Vbat/1
  AC/DC Converter/5(IQ) -> [IQ]
  5 Charging Stations/4(Voltage) -> [Vbat]
  [Ibat] -> Scope Ibat/1
  [Vabc2] -> Mux3/1, 3-Phase Voltage & Current/1, "Power (3ph, Instantaneous)"/1
  5 Charging Stations/2(SOC) -> [SOC]
  5 Charging Stations/1(to_workspace) -> To Workspace/1
  "Power (3ph, Instantaneous)"/1 -> Mux4/1, Active Power/1
  [VDC] -> To Workspace3/1, DC Voltage/1
  Mux4/1 -> To Workspace2/1
  "Power (3ph, Instantaneous)"/2 -> Scope Reactive Power/1, Mux4/2
  Mux3/1 -> To Workspace1/1
  MovingRMSFaultDetect2/2(Ibat_ref) -> Mux1/2, ControlFault2/2, GotoV2G_FaultDetect/1
  From11/1 -> MovingRMSFaultDetect2/1(Vabc)
  From12/1 -> MovingRMSFaultDetect2/2(Iabc)
  MovingRMSFaultDetect2/1(Vrms) -> Mux1/1, ControlFault2/1
  ConstantG2V/1 -> [Ibat_ref2]
  Mux1/1 -> ToWorkspaceFaultDetect/1
  From2/1 -> V2G_Gajduk/1(Vabc)
  Constant5/1 -> V2G_Gajduk/2(f_grid)
  Mux2/1 -> ToWorkspaceGajduk/1
  V2G_Gajduk/2(Ibat_ref) -> Mux2/2, ControlFreq2/2, GotoV2G_Gajduk/1
  V2G_Gajduk/1(delta_f) -> Mux2/1, ControlFreq2/1, Frequency Deviation2/1
  connections:
  AC/DC Converter/LConn2 -- Series RLC Branch7/RConn1
  Series RLC Branch/RConn1 -- Series RLC Branch6/LConn1 -- Series RLC Branch11/LConn1
  AC/DC Converter/RConn2 -- 5 Charging Stations/LConn2 -- Series RLC Branch5/RConn1
  Series RLC Branch4/LConn1 -- Series RLC Branch8/LConn1 -- Series RLC Branch2/RConn1
  A/RConn1 -- Three-Phase V-I Measurement/LConn1
  B/RConn1 -- Three-Phase V-I Measurement/LConn2
  AC/DC Converter/RConn1 -- 5 Charging Stations/LConn1 -- Series RLC Branch5/LConn1
  AC/DC Converter/LConn3 -- Series RLC Branch8/RConn1
  AC/DC Converter/LConn1 -- Series RLC Branch6/RConn1
  C/RConn1 -- Three-Phase V-I Measurement/LConn3
  Series RLC Branch3/RConn1 -- Series RLC Branch11/RConn1 -- Series RLC Branch4/RConn1
  Series RLC Branch/LConn1 -- Three-Phase V-I Measurement/RConn1
  Series RLC Branch1/LConn1 -- Three-Phase V-I Measurement/RConn2
  Series RLC Branch3/LConn1 -- Series RLC Branch1/RConn1 -- Series RLC Branch7/LConn1
  Series RLC Branch2/LConn1 -- Three-Phase V-I Measurement/RConn3

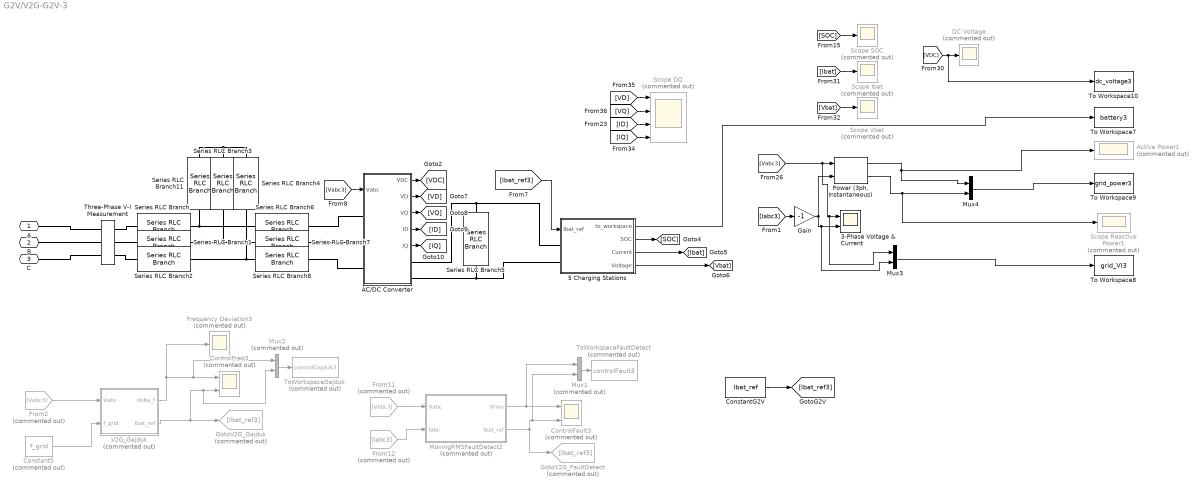
== system G2V/V2G-G2V-3 ==
  3-Phase Voltage & Current : Scope  NumInputPorts=2
  5 Charging Stations : Subsystem
  AC/DC Converter : Subsystem
  Active Power1 : Scope  Commented=on
  Constant5 : Constant  Commented=on  Value=f_grid
  ConstantG2V : Constant  Value=Ibat_ref
  ControlFault3 : Scope  Commented=on  NumInputPorts=2
  ControlFreq3 : Scope  Commented=on  NumInputPorts=2
  DC Voltage : Scope  Commented=on
  Frequency Deviation3 : Scope  Commented=on
  From11 : From  Commented=on  GotoTag=Vabc3  TagVisibility=global
  From12 : From  Commented=on  GotoTag=Iabc3  TagVisibility=global
  From2 : From  Commented=on  GotoTag=Vabc3  TagVisibility=global
  Gain : Gain  Gain=-1
  GotoV2G_FaultDetect : Goto  Commented=on  GotoTag=Ibat_ref3
  GotoV2G_Gajduk : Goto  Commented=on  GotoTag=Ibat_ref3
  MovingRMSFaultDetect2 : Subsystem  Commented=on
  Mux1 : Mux  Commented=on  Inputs=2
  Mux2 : Mux  Commented=on  Inputs=2
  Mux3 : Mux  Inputs=2
  Mux4 : Mux  Inputs=2
  "Power (3ph, Instantaneous)" : powerlib_meascontrol/Measurements/Power (3ph, Instantaneous)
      settings: SourceProductName=Simscape Power Systems
  Scope DQ : Scope  Commented=on  NumInputPorts=4
  Scope Ibat : Scope  Commented=on
  Scope Reactive Power1 : Scope  Commented=on
  Scope SOC : Scope  Commented=on
  Scope Vbat : Scope  Commented=on
  Series RLC Branch : powerlib/Elements/Series RLC Branch  LConnTagsString=__new0  RConnTagsString=__new0  BranchType=L  Resistance=1  Inductance=Lgrid  SetiL0=off  InitialCurrent=0  Capacitance=1e-6  Setx0=off  InitialVoltage=0  Measurements=None
  Series RLC Branch1 : powerlib/Elements/Series RLC Branch  LConnTagsString=__new0  RConnTagsString=__new0  BranchType=L  Resistance=1  Inductance=Lgrid  SetiL0=off  InitialCurrent=0  Capacitance=1e-6  Setx0=off  InitialVoltage=0  Measurements=None
  Series RLC Branch11 : powerlib/Elements/Series RLC Branch  LConnTagsString=__new0  RConnTagsString=__new0  BranchType=RC  Resistance=Rd  Inductance=Lbuckboost  SetiL0=off  InitialCurrent=0  Capacitance=Cf  Setx0=off  InitialVoltage=0  Measurements=None
  Series RLC Branch2 : powerlib/Elements/Series RLC Branch  LConnTagsString=__new0  RConnTagsString=__new0  BranchType=L  Resistance=1  Inductance=Lgrid  SetiL0=off  InitialCurrent=0  Capacitance=1e-6  Setx0=off  InitialVoltage=0  Measurements=None
  Series RLC Branch3 : powerlib/Elements/Series RLC Branch  LConnTagsString=__new0  RConnTagsString=__new0  BranchType=RC  Resistance=Rd  Inductance=Lbuckboost  SetiL0=off  InitialCurrent=0  Capacitance=Cf  Setx0=off  InitialVoltage=0  Measurements=None
  Series RLC Branch4 : powerlib/Elements/Series RLC Branch  LConnTagsString=__new0  RConnTagsString=__new0  BranchType=RC  Resistance=Rd  Inductance=Lbuckboost  SetiL0=off  InitialCurrent=0  Capacitance=Cf  Setx0=off  InitialVoltage=0  Measurements=None
  Series RLC Branch5 : powerlib/Elements/Series RLC Branch  LConnTagsString=__new0  RConnTagsString=__new0  BranchType=C  Resistance=R_Vdc  Inductance=1e-3  SetiL0=off  InitialCurrent=0  Capacitance=C_Vdc  Setx0=on  InitialVoltage=V0_Vdc  Measurements=None
  Series RLC Branch6 : powerlib/Elements/Series RLC Branch  LConnTagsString=__new0  RConnTagsString=__new0  BranchType=L  Resistance=1  Inductance=Linv  SetiL0=off  InitialCurrent=0  Capacitance=1e-6  Setx0=off  InitialVoltage=0  Measurements=None
  Series RLC Branch7 : powerlib/Elements/Series RLC Branch  LConnTagsString=__new0  RConnTagsString=__new0  BranchType=L  Resistance=1  Inductance=Linv  SetiL0=off  InitialCurrent=0  Capacitance=1e-6  Setx0=off  InitialVoltage=0  Measurements=None
  Series RLC Branch8 : powerlib/Elements/Series RLC Branch  LConnTagsString=__new0  RConnTagsString=__new0  BranchType=L  Resistance=1  Inductance=Linv  SetiL0=off  InitialCurrent=0  Capacitance=1e-6  Setx0=off  InitialVoltage=0  Measurements=None
  Three-Phase V-I Measurement : powerlib/Measurements/Three-Phase V-I Measurement  VoltageMeasurement=phase-to-ground  SetLabelV=on  LabelV=Vabc3  Vpu=off  VpuLL=off  CurrentMeasurement=yes  SetLabelI=on  LabelI=Iabc3  Ipu=off  Pbase=100e6  Vbase=500e3  OutputType=Complex  PhasorSimulation=off  PSBequivalent=0
  To Workspace10 : ToWorkspace  VariableName=dc_voltage3  SaveFormat=Timeseries  SampleTime=-1
  To Workspace7 : ToWorkspace  VariableName=battery3  SaveFormat=Timeseries  SampleTime=-1
  To Workspace8 : ToWorkspace  VariableName=grid_VI3  SaveFormat=Timeseries  SampleTime=-1
  To Workspace9 : ToWorkspace  VariableName=grid_power3  SaveFormat=Timeseries  SampleTime=-1
  ToWorkspaceFaultDetect : ToWorkspace  Commented=on  VariableName=controlFault3  SaveFormat=Timeseries  SampleTime=-1
  ToWorkspaceGajduk : ToWorkspace  Commented=on  VariableName=controlGajduk3  SaveFormat=Timeseries  SampleTime=-1
  V2G_Gajduk : Subsystem  Commented=on
  A : PMIOPort  Port=1  Side=Left
  B : PMIOPort  Port=2  Side=Left
  C : PMIOPort  Port=3  Side=Left
  wires:
  AC/DC Converter/3(VQ) -> [VQ]
  AC/DC Converter/4(ID) -> [ID]
  Gain/1 -> Mux3/2, 3-Phase Voltage & Current/2, "Power (3ph, Instantaneous)"/2
  AC/DC Converter/5(IQ) -> [IQ]
  [VQ] -> Scope DQ/2
  AC/DC Converter/2(VD) -> [VD]
  5 Charging Stations/4(Voltage) -> [Vbat]
  [Vabc3] -> AC/DC Converter/1(Vabc)
  [VD] -> Scope DQ/1
  [Ibat] -> Scope Ibat/1
  AC/DC Converter/1(VDC) -> [VDC]
  [Vabc3] -> Mux3/1, 3-Phase Voltage & Current/1, "Power (3ph, Instantaneous)"/1
  [IQ] -> Scope DQ/4
  5 Charging Stations/2(SOC) -> [SOC]
  [Vbat] -> Scope Vbat/1
  [Iabc3] -> Gain/1
  [SOC] -> Scope SOC/1
  [ID] -> Scope DQ/3
  [Ibat_ref3] -> 5 Charging Stations/1(Ibat_ref)
  5 Charging Stations/3(Current) -> [Ibat]
  [VDC] -> To Workspace10/1, DC Voltage/1
  Mux4/1 -> To Workspace9/1
  "Power (3ph, Instantaneous)"/1 -> Active Power1/1, Mux4/1
  5 Charging Stations/1(to_workspace) -> To Workspace7/1
  "Power (3ph, Instantaneous)"/2 -> Scope Reactive Power1/1, Mux4/2
  Mux3/1 -> To Workspace8/1
  From2/1 -> V2G_Gajduk/1(Vabc)
  Mux2/1 -> ToWorkspaceGajduk/1
  Constant5/1 -> V2G_Gajduk/2(f_grid)
  V2G_Gajduk/1(delta_f) -> Mux2/1, ControlFreq3/1, Frequency Deviation3/1
  V2G_Gajduk/2(Ibat_ref) -> Mux2/2, ControlFreq3/2, GotoV2G_Gajduk/1
  Mux1/1 -> ToWorkspaceFaultDetect/1
  From12/1 -> MovingRMSFaultDetect2/2(Iabc)
  MovingRMSFaultDetect2/1(Vrms) -> Mux1/1, ControlFault3/1
  From11/1 -> MovingRMSFaultDetect2/1(Vabc)
  MovingRMSFaultDetect2/2(Ibat_ref) -> Mux1/2, ControlFault3/2, GotoV2G_FaultDetect/1
  ConstantG2V/1 -> [Ibat_ref3]
  connections:
  Series RLC Branch/LConn1 -- Three-Phase V-I Measurement/RConn1
  A/RConn1 -- Three-Phase V-I Measurement/LConn1
  AC/DC Converter/LConn3 -- Series RLC Branch8/RConn1
  5 Charging Stations/LConn2 -- AC/DC Converter/RConn2 -- Series RLC Branch5/RConn1
  Series RLC Branch11/RConn1 -- Series RLC Branch3/RConn1 -- Series RLC Branch4/RConn1
  Series RLC Branch3/LConn1 -- Series RLC Branch1/RConn1 -- Series RLC Branch7/LConn1
  AC/DC Converter/LConn1 -- Series RLC Branch6/RConn1
  Series RLC Branch2/LConn1 -- Three-Phase V-I Measurement/RConn3
  AC/DC Converter/LConn2 -- Series RLC Branch7/RConn1
  Series RLC Branch5/LConn1 -- AC/DC Converter/RConn1 -- 5 Charging Stations/LConn1
  B/RConn1 -- Three-Phase V-I Measurement/LConn2
  C/RConn1 -- Three-Phase V-I Measurement/LConn3
  Series RLC Branch4/LConn1 -- Series RLC Branch8/LConn1 -- Series RLC Branch2/RConn1
  Series RLC Branch6/LConn1 -- Series RLC Branch/RConn1 -- Series RLC Branch11/LConn1
  Series RLC Branch1/LConn1 -- Three-Phase V-I Measurement/RConn2

== system G2V/V2G-G2V-1/5 Charging Stations ==
  Ibat_ref : Inport
  Charging Station1 : Subsystem
  Charging Station10 : Subsystem  Commented=on
  Charging Station2 : Subsystem
  Charging Station3 : Subsystem
  Charging Station4 : Subsystem
  Charging Station5 : Subsystem
  Charging Station6 : Subsystem  Commented=on
  Charging Station7 : Subsystem  Commented=on
  Charging Station8 : Subsystem  Commented=on
  Charging Station9 : Subsystem  Commented=on
  VDC+ : PMIOPort  Port=1  Side=Left
  VDC- : PMIOPort  Port=2  Side=Left
  to_workspace : Outport
  SOC : Outport  Port=2
  Current : Outport  Port=3
  Voltage : Outport  Port=4
  wires:
  Charging Station1/3(Current) -> Current/1
  Charging Station1/2(SOC) -> SOC/1
  Charging Station1/4(Voltage) -> Voltage/1
  Charging Station1/1(to_workspace) -> to_workspace/1
  Ibat_ref/1 -> Charging Station10/1(Ibat_ref), Charging Station9/1(Ibat_ref), Charging Station8/1(Ibat_ref), Charging Station7/1(Ibat_ref), Charging Station6/1(Ibat_ref), Charging Station5/1(Ibat_ref), Charging Station4/1(Ibat_ref), Charging Station3/1(Ibat_ref), Charging Station2/1(Ibat_ref), Charging Station1/1(Ibat_ref)
  connections:
  Charging Station9/LConn2 -- Charging Station10/LConn2 -- VDC-/RConn1 -- Charging Station1/LConn2 -- Charging Station2/LConn2 -- Charging Station3/LConn2 -- Charging Station4/LConn2 -- Charging Station5/LConn2 -- Charging Station6/LConn2 -- Charging Station7/LConn2 -- Charging Station8/LConn2
  Charging Station9/LConn1 -- Charging Station10/LConn1 -- Charging Station1/LConn1 -- VDC+/RConn1 -- Charging Station2/LConn1 -- Charging Station3/LConn1 -- Charging Station4/LConn1 -- Charging Station5/LConn1 -- Charging Station6/LConn1 -- Charging Station7/LConn1 -- Charging Station8/LConn1
